simulink model "simulink_collect_data_NN"  (R2022b)
settings: Solver=ode4  StartTime=0.0  StopTime=10  FixedStep=0.001  RelTol=1e-3
values from neighbouring files (symbols this model uses):
  thetastartdelta = rand * 0.6 - 0.3    [collect_data_NN.m]
  xstartdelta = rand - 0.5    [collect_data_NN.m]
undefined symbols (not defined in the file or in its folder): A, aa, B, bb, C, cc, D, dd, ee, ff, KK, mm, nn, thetastart, xstart
settings Model: Creator=manzand  LastModifiedBy=Wolfgang
settings SolverCC: AlgebraicLoopSolver=TrustRegion
settings DataIOCC: ReturnWorkspaceOutputs=off
settings DebuggingCC: UnconnectedInputMsg=warning  UnconnectedOutputMsg=warning  UnconnectedLineMsg=warning  SFMachineParentedDataDiag=warning  ArithmeticOperatorsInVariantConditions=warning
settings ModelReferenceCC: EnableRefExpFcnMdlSchedulingChecks=on
settings SFSimCC: SimUseLocalCustomCode=off  CustomCodeUndefinedFunction=UseInterfaceOnly
settings RTWCC: RTWUseLocalCustomCode=off
settings CodeAppCC: StateflowObjectComments=on

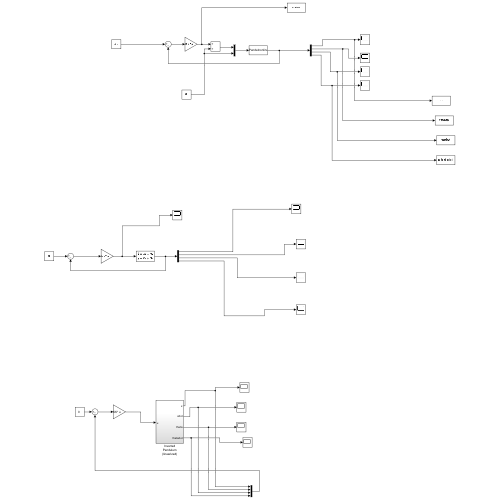
[thumbnail: Simulink's stored preview of the top-level diagram]
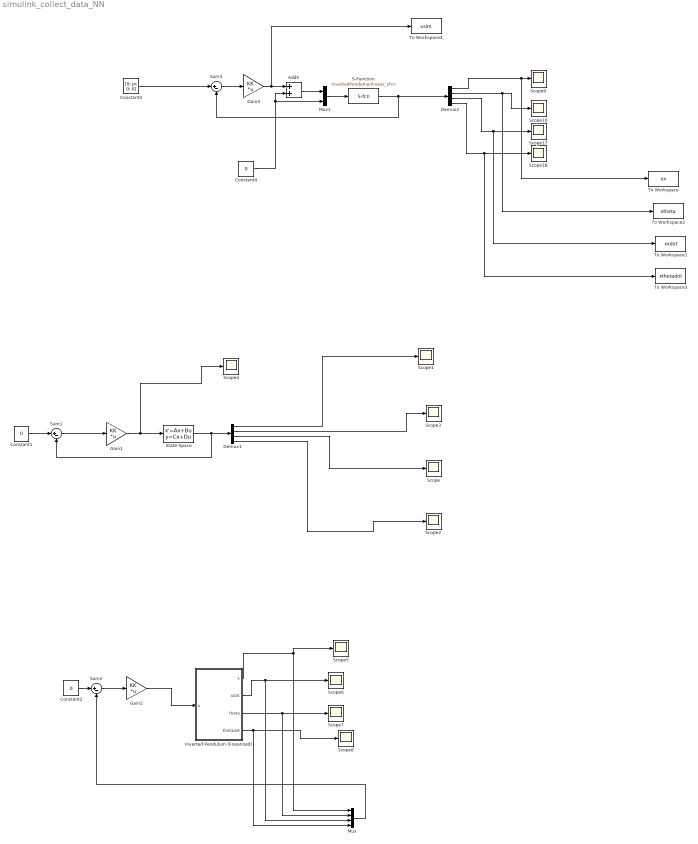
== system simulink_collect_data_NN ==
  Add5 : Sum
  Constant1 : Constant  Value=0
  Constant2 : Constant  Value=0
  Constant3 : Constant  Value=[0; pi; 0; 0]
  Constant4 : Constant  Value=0
  Demux1 : Demux
  Demux2 : Demux
  Gain1 : Gain  Gain=KK  Multiplication=Matrix(K*u)
  Gain2 : Gain  Gain=KK  Multiplication=Matrix(K*u)
  Gain3 : Gain  Gain=KK  Multiplication=Matrix(K*u)
  Inverted Pendulum (linearized) : Subsystem
  Mux : Mux
  Mux1 : Mux  Inputs=2
  S-Function : S-Function  FunctionName=invertedPendelnonlinear_sfcn  Parameters=xstart+xstartdelta; thetastart+thetastartdelta; 0; 0  SFunctionDeploymentMode=off  EnableBusSupport=off
  Scope{,1..10,17..18} (13 alike) : Scope
  State-Space : StateSpace  A=A  B=B  C=C  D=D  InitialCondition=[xstart; thetastart; 0;0]
  Sum1 : Sum  Inputs=|+-
  Sum2 : Sum  Inputs=|+-
  Sum3 : Sum  Inputs=|+-
  To Workspace : ToWorkspace  VariableName=xx  SampleTime=0.005
      settings: Decimation=2  Save2DSignal=2-D array (concatenate along first dimension)
  To Workspace1 : ToWorkspace  VariableName=xxdot  SampleTime=0.005
      settings: Decimation=2  Save2DSignal=2-D array (concatenate along first dimension)
  To Workspace2 : ToWorkspace  VariableName=xtheta  SampleTime=0.005
      settings: Decimation=2  Save2DSignal=2-D array (concatenate along first dimension)
  To Workspace3 : ToWorkspace  VariableName=xthetadot  SampleTime=0.005
      settings: Decimation=2  Save2DSignal=2-D array (concatenate along first dimension)
  To Workspace4 : ToWorkspace  VariableName=usim  SampleTime=0.005
      settings: Decimation=2  Save2DSignal=2-D array (concatenate along first dimension)
  wires:
  Demux1/1 -> Scope1/1
  State-Space/1 -> Sum1/2, Demux1/1
  Constant1/1 -> Sum1/1
  Sum1/1 -> Gain1/1
  Gain1/1 -> State-Space/1, Scope4/1
  Demux1/3 -> Scope/1
  Demux1/2 -> Scope3/1
  Gain2/1 -> Inverted Pendulum (linearized)/1(u)
  Mux/1 -> Sum2/2
  Sum2/1 -> Gain2/1
  Constant2/1 -> Sum2/1
  Inverted Pendulum (linearized)/4(thetadot) -> Mux/4, Scope8/1
  Inverted Pendulum (linearized)/3(theta) -> Mux/2, Scope7/1
  Inverted Pendulum (linearized)/2(xdot) -> Mux/3, Scope6/1
  Inverted Pendulum (linearized)/1(x) -> Mux/1, Scope5/1
  Demux1/4 -> Scope2/1
  Demux2/3 -> To Workspace1/1, Scope17/1
  Demux2/4 -> To Workspace3/1, Scope18/1
  Demux2/1 -> Scope9/1, To Workspace/1
  Demux2/2 -> To Workspace2/1, Scope10/1
  S-Function/1 -> Sum3/2, Demux2/1
  Gain3/1 -> To Workspace4/1, Add5/1
  Add5/1 -> Mux1/1
  Mux1/1 -> S-Function/1
  Sum3/1 -> Gain3/1
  Constant3/1 -> Sum3/1
  Constant4/1 -> Mux1/2, Add5/2

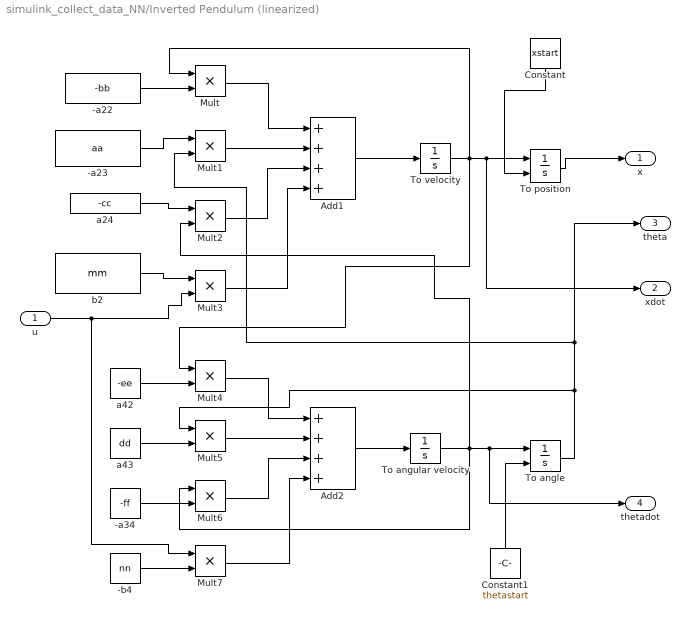
== system simulink_collect_data_NN/Inverted Pendulum (linearized) ==
  u : Inport
  -a22 : Constant  Value=-bb
  -a23 : Constant  Value=aa
  -a34 : Constant  Value=-ff
  -b4 : Constant  Value=nn
  Add1 : Sum  Inputs=++++
  Add2 : Sum  Inputs=++++
  Constant : Constant  Value=xstart
  Constant1 : Constant  Value=thetastart
  Mult{,1..7} (8 alike) : Product  Inputs=**
  To angle : Integrator  InitialConditionSource=external  InitialCondition=1.5
  To angular velocity : Integrator
  To position : Integrator  InitialConditionSource=external  InitialCondition=1
  To velocity : Integrator
  a24 : Constant  Value=-cc
  a42 : Constant  Value=-ee
  a43 : Constant  Value=dd
  b2 : Constant  Value=mm
  x : Outport  VectorParamsAs1DForOutWhenUnconnected=off
  xdot : Outport  Port=2  VectorParamsAs1DForOutWhenUnconnected=off
  theta : Outport  Port=3  VectorParamsAs1DForOutWhenUnconnected=off
  thetadot : Outport  Port=4  VectorParamsAs1DForOutWhenUnconnected=off
  wires:
  -a22/1 -> Mult/2
  Add2/1 -> To angular velocity/1
  -a34/1 -> Mult6/2
  -b4/1 -> Mult7/2
  Mult6/1 -> Add2/3
  Mult3/1 -> Add1/4
  Mult1/1 -> Add1/2
  Add1/1 -> To velocity/1
  b2/1 -> Mult3/1
  To angular velocity/1 -> Mult6/1, Mult2/2, thetadot/1, To angle/1
  -a23/1 -> Mult1/1
  To velocity/1 -> Mult4/1, Mult/1, xdot/1, To position/1
  To angle/1 -> theta/1, Mult1/2, Mult5/1
  Mult7/1 -> Add2/4
  a43/1 -> Mult5/2
  Mult4/1 -> Add2/1
  Mult2/1 -> Add1/3
  u/1 -> Mult7/1, Mult3/2
  a42/1 -> Mult4/2
  Mult/1 -> Add1/1
  Mult5/1 -> Add2/2
  a24/1 -> Mult2/1
  To position/1 -> x/1
  Constant1/1 -> To angle/2
  Constant/1 -> To position/2
